simulink model "Simulation"  (Simulink 6.0)
settings: Solver=ode3  StartTime=0.0  StopTime=10  FixedStep=5e-3  RelTol=5e-3
values from neighbouring files (symbols this model uses):
  s = sqrt(1-rot(1,1)-rot(2,2)+rot(3,3))*2    [rot_to_quat2.m]
undefined symbols (not defined in the file or in its folder): sigbuilder_block
libraries: simulink x30, mblibv1 x15, aerolibtransform2 x4, vrlib x1
(part 2 of 2)

== system Simulation/Subsystem/Gestion Dynamique/Calcul orientation ==
  Erreur orientation : Inport  Port=1  LatchInput=off
  Orientation : Inport  Port=2  LatchInput=off
  Constant : Constant  Value=0
  Constant1 : Constant  Value=0
  Constant2 : Constant  Value=0
  Demux : Demux  Outputs=3
  Mux : Mux  Inputs=6
  Product : Product  RndMeth=Zero
  Product1 : Product  Multiplication=Matrix(*)  RndMeth=Zero
  Quaternion 2 AngleVecteur : Subsystem
  Quaternions to  Direction Cosine Matrix : aerolibtransform2/Quaternions to  Direction Cosine Matrix
  Reshape5 : simulink/Math Operations/Reshape  OutputDimensionality=1-D array  OutputDimensions=[1,1]
  Scope : Scope  NumInputPorts=2
      settings: YMin=-5~-5  YMax=5~5  SaveName=ScopeData11
  Ordres orientation : Outport
      settings: BusObject=perturbations
  wires:
  Mux/1 -> Reshape5/1
  Reshape5/1 -> Ordres orientation/1
  Constant/1 -> Mux/1
  Constant1/1 -> Mux/2
  Constant2/1 -> Mux/3
  Erreur orientation/1 -> Quaternion 2 AngleVecteur/1(Quaternion)
  Demux/1 -> Mux/4
  Demux/2 -> Mux/5
  Demux/3 -> Mux/6
  Product/1 -> Scope/2, Product1/2
  Quaternion 2 AngleVecteur/2(Vecteur) -> Product/2
  Quaternion 2 AngleVecteur/1(Angle) -> Product/1, Scope/1
  Quaternions to  Direction Cosine Matrix/1 -> Product1/1
  Product1/1 -> Demux/1
  Orientation/1 -> Quaternions to  Direction Cosine Matrix/1

== system Simulation/Subsystem/Gestion Dynamique/PID Attitude ==
  Entrée : Inport  Port=1  LatchInput=off
  Derivative : Derivative
  Derivative1 : Derivative
  Derivative2 : Derivative
  Gain : Gain  Gain=kp
  Gain1 : Gain  Gain=kd
  Gain2 : Gain  Gain=ki
  Gain3 : Gain  Gain=kdd
  Integrator : Integrator
  Reshape : simulink/Math Operations/Reshape  OutputDimensionality=1-D array  OutputDimensions=[1,1]
  Sum : Sum  Inputs=++++
  Sortie : Outport
      settings: BusObject=perturbations
  wires:
  Entrée/1 -> Gain/1
  Gain/1 -> Sum/2, Gain1/1, Gain2/1, Gain3/1
  Derivative/1 -> Sum/1
  Integrator/1 -> Sum/3
  Gain2/1 -> Integrator/1
  Gain1/1 -> Derivative/1
  Sum/1 -> Reshape/1
  Gain3/1 -> Derivative1/1
  Derivative1/1 -> Derivative2/1
  Derivative2/1 -> Sum/4
  Reshape/1 -> Sortie/1

== system Simulation/Subsystem/Gestion Dynamique/PID Position ==
  Entrée : Inport  Port=1  LatchInput=off
  Derivative : Derivative
  Derivative1 : Derivative
  Derivative2 : Derivative
  Gain : Gain  Gain=kp
  Gain1 : Gain  Gain=kd
  Gain2 : Gain  Gain=ki
  Gain3 : Gain  Gain=kdd
  Integrator : Integrator
  Reshape : simulink/Math Operations/Reshape  OutputDimensionality=1-D array  OutputDimensions=[1,1]
  Saturation : Saturate  UpperLimit=0.1  LowerLimit=-0.1
  Sum : Sum  Inputs=++++
  Sortie : Outport
      settings: BusObject=perturbations
  wires:
  Entrée/1 -> Gain/1
  Gain/1 -> Sum/2, Gain1/1, Gain2/1, Gain3/1
  Derivative/1 -> Sum/1
  Integrator/1 -> Saturation/1
  Gain2/1 -> Integrator/1
  Gain1/1 -> Derivative/1
  Sum/1 -> Reshape/1
  Gain3/1 -> Derivative1/1
  Derivative1/1 -> Derivative2/1
  Derivative2/1 -> Sum/4
  Reshape/1 -> Sortie/1
  Saturation/1 -> Sum/3

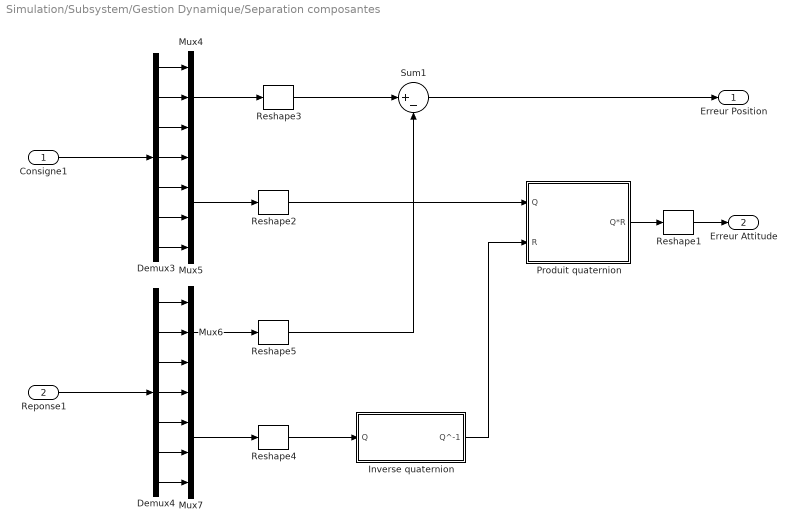
== system Simulation/Subsystem/Gestion Dynamique/Separation composantes ==
  Consigne1 : Inport  Port=1  LatchInput=off
  Reponse1 : Inport  Port=2  LatchInput=off
  Demux3 : Demux  Outputs=7
  Demux4 : Demux  Outputs=7
  Inverse quaternion : Subsystem
  Mux4 : Mux  Inputs=3
  Mux5 : Mux
  Mux6 : Mux  Inputs=3
  Mux7 : Mux
  Produit quaternion : Subsystem
  Reshape{1..5} (5 alike) : simulink/Math Operations/Reshape  OutputDimensionality=1-D array  OutputDimensions=[1,1]
  Sum1 : Sum  Inputs=|+-
  Erreur Position : Outport
      settings: BusObject=perturbations
  Erreur Attitude : Outport  Port=2
      settings: BusObject=perturbations
  wires:
  Consigne1/1 -> Demux3/1
  Demux3/4 -> Mux5/1
  Demux3/5 -> Mux5/2
  Demux3/6 -> Mux5/3
  Demux3/7 -> Mux5/4
  Demux3/3 -> Mux4/3
  Demux3/2 -> Mux4/2
  Demux3/1 -> Mux4/1
  Mux5/1 -> Reshape2/1
  Mux4/1 -> Reshape3/1
  Demux4/4 -> Mux7/1
  Demux4/5 -> Mux7/2
  Demux4/6 -> Mux7/3
  Demux4/7 -> Mux7/4
  Demux4/3 -> Mux6/3
  Demux4/2 -> Mux6/2
  Demux4/1 -> Mux6/1
  Reponse1/1 -> Demux4/1
  Mux7/1 -> Reshape4/1
  Mux6/1 -> Reshape5/1
  Reshape3/1 -> Sum1/1
  Reshape5/1 -> Sum1/2
  Sum1/1 -> Erreur Position/1
  Reshape4/1 -> Inverse quaternion/1(Q)
  Reshape2/1 -> Produit quaternion/1(Q)
  Inverse quaternion/1(Q^-1) -> Produit quaternion/2(R)
  Produit quaternion/1(Q*R) -> Reshape1/1
  Reshape1/1 -> Erreur Attitude/1

== system Simulation/Subsystem/Gestion Dynamique/Separation composantes1 ==
  Entree : Inport  Port=1  LatchInput=off
  Demux1 : Demux  Outputs=7
  Mux : Mux  Inputs=3
  Mux1 : Mux
  Reshape : simulink/Math Operations/Reshape  OutputDimensionality=1-D array  OutputDimensions=[1,1]
  Reshape1 : simulink/Math Operations/Reshape  OutputDimensionality=1-D array  OutputDimensions=[1,1]
  Position : Outport
      settings: BusObject=perturbations
  Orientation : Outport  Port=2
      settings: BusObject=perturbations
  wires:
  Entree/1 -> Demux1/1
  Demux1/4 -> Mux1/1
  Demux1/5 -> Mux1/2
  Demux1/6 -> Mux1/3
  Demux1/7 -> Mux1/4
  Demux1/3 -> Mux/3
  Demux1/2 -> Mux/2
  Demux1/1 -> Mux/1
  Mux1/1 -> Reshape/1
  Mux/1 -> Reshape1/1
  Reshape/1 -> Orientation/1
  Reshape1/1 -> Position/1

== system Simulation/Subsystem/Gestion Dynamique/Sommation ordres ==
  Ordres position : Inport  Port=1  LatchInput=off
  Ordres orientation : Inport  Port=2  LatchInput=off
  Sum : Sum
  Ordres : Outport
      settings: BusObject=perturbations
  wires:
  Ordres orientation/1 -> Sum/2
  Sum/1 -> Ordres/1
  Ordres position/1 -> Sum/1

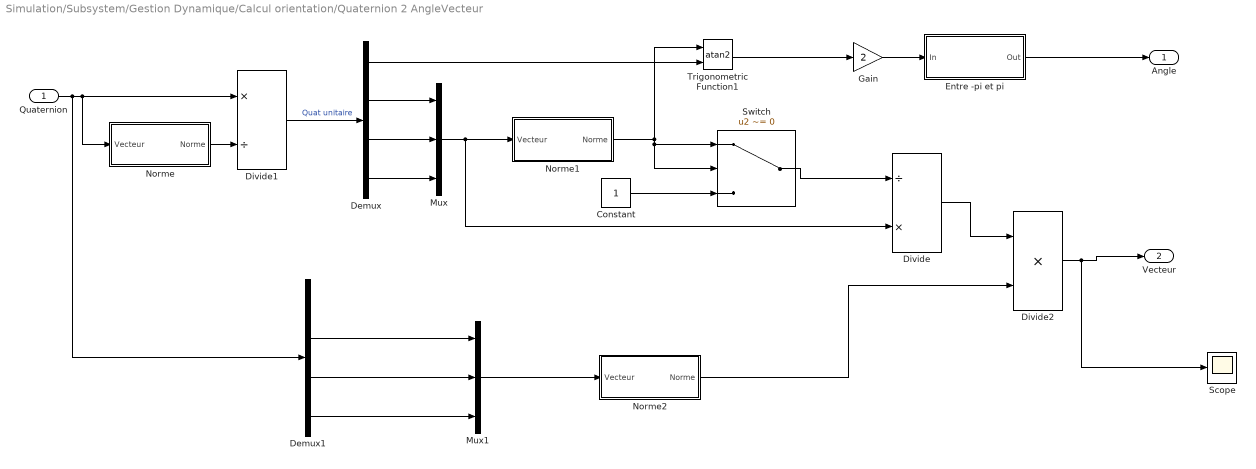
== system Simulation/Subsystem/Gestion Dynamique/Calcul orientation/Quaternion 2 AngleVecteur ==
  Quaternion : Inport  Port=1  LatchInput=off
  Constant : Constant
  Demux : Demux
  Demux1 : Demux
  Divide : Product  Inputs=/*  OutScaling=2^-10
  Divide1 : Product  Inputs=*/  OutScaling=2^-10
  Divide2 : Product  Inputs=**  OutScaling=2^-10
  Entre -pi et pi : Subsystem  mask{ordre=2}
  Gain : Gain  Gain=2
  Mux : Mux  Inputs=3
  Mux1 : Mux  Inputs=3
  Norme : Subsystem  mask{ordre=2}
      mask Display: text(0.3,0.5,strcat('Norme',get_param(gcb, 'ordre')));
  Norme1 : Subsystem  mask{ordre=2}
      mask Display: text(0.3,0.5,strcat('Norme',get_param(gcb, 'ordre')));
  Norme2 : Subsystem  mask{ordre=2}
      mask Display: text(0.3,0.5,strcat('Norme',get_param(gcb, 'ordre')));
  Scope : Scope
      settings: SaveName=ScopeData10
  Switch : Switch  Criteria=u2 ~= 0
  Trigonometric Function1 : Trigonometry  Operator=atan2
  Angle : Outport
  Vecteur : Outport  Port=2
  wires:
  Quaternion/1 -> Divide1/1, Norme/1(Vecteur), Demux1/1
  Trigonometric Function1/1 -> Gain/1
  Norme/1(Norme) -> Divide1/2
  Divide1/1 -> Demux/1  "Quat unitaire"
  Mux/1 -> Norme1/1(Vecteur), Divide/2
  Demux/2 -> Mux/1
  Demux/3 -> Mux/2
  Demux/4 -> Mux/3
  Norme1/1(Norme) -> Trigonometric Function1/1, Switch/2, Switch/1
  Demux/1 -> Trigonometric Function1/2
  Switch/1 -> Divide/1
  Constant/1 -> Switch/3
  Entre -pi et pi/1(Out) -> Angle/1
  Gain/1 -> Entre -pi et pi/1(In)
  Demux1/2 -> Mux1/1
  Demux1/3 -> Mux1/2
  Demux1/4 -> Mux1/3
  Mux1/1 -> Norme2/1(Vecteur)
  Divide/1 -> Divide2/1
  Norme2/1(Norme) -> Divide2/2
  Divide2/1 -> Vecteur/1, Scope/1

== system Simulation/Subsystem/Gestion Dynamique/Separation composantes/Inverse quaternion ==
  Q : Inport  Port=1  LatchInput=off
  Gain : Gain  Gain=[1 -1 -1 -1]
  Q^-1 : Outport
  wires:
  Q/1 -> Gain/1
  Gain/1 -> Q^-1/1

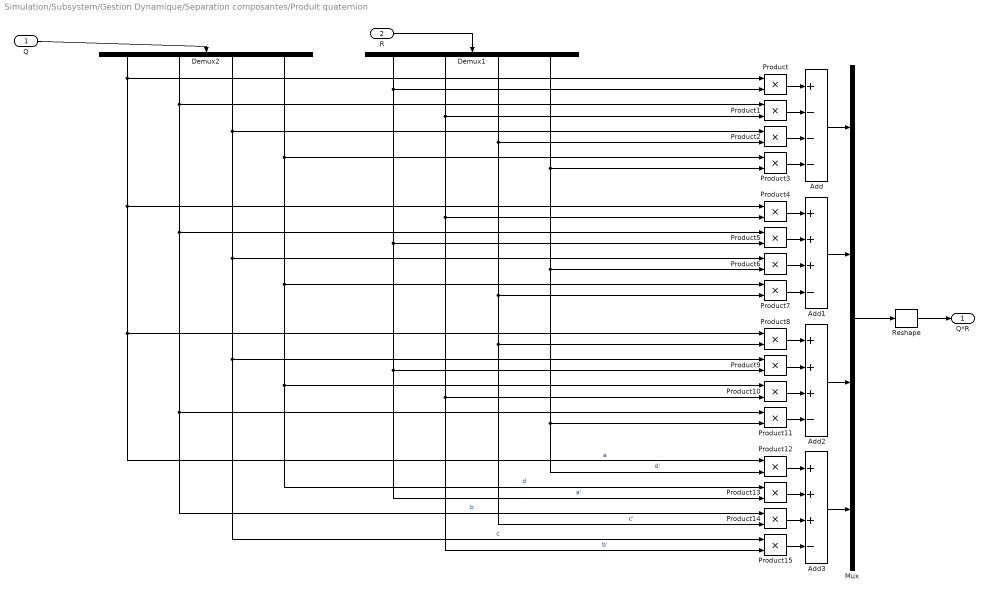
== system Simulation/Subsystem/Gestion Dynamique/Separation composantes/Produit quaternion ==
  Q : Inport  Port=1  LatchInput=off
  R : Inport  Port=2  LatchInput=off
  Add : Sum  Inputs=+---  OutScaling=2^-10
  Add1 : Sum  Inputs=+++-  OutScaling=2^-10
  Add2 : Sum  Inputs=+++-  OutScaling=2^-10
  Add3 : Sum  Inputs=+++-  OutScaling=2^-10
  Demux1 : Demux  Orientation=down
  Demux2 : Demux  Orientation=down
  Mux : Mux
  Product{,1..15} (16 alike) : Product  RndMeth=Zero
  Reshape : simulink/Math Operations/Reshape  OutputDimensionality=1-D array  OutputDimensions=[1,1]
  Q*R : Outport
  wires:
  R/1 -> Demux1/1
  Q/1 -> Demux2/1
  Mux/1 -> Reshape/1
  Reshape/1 -> Q*R/1
  Demux2/1 -> Product/1, Product4/1, Product8/1, Product12/1  "a"
  Add/1 -> Mux/1
  Add1/1 -> Mux/2
  Add2/1 -> Mux/3
  Add3/1 -> Mux/4
  Product3/1 -> Add/4
  Product2/1 -> Add/3
  Product1/1 -> Add/2
  Product/1 -> Add/1
  Product7/1 -> Add1/4
  Product6/1 -> Add1/3
  Product5/1 -> Add1/2
  Product4/1 -> Add1/1
  Product11/1 -> Add2/4
  Product10/1 -> Add2/3
  Product9/1 -> Add2/2
  Product8/1 -> Add2/1
  Product15/1 -> Add3/4
  Product14/1 -> Add3/3
  Product13/1 -> Add3/2
  Product12/1 -> Add3/1
  Demux2/2 -> Product1/1, Product5/1, Product11/1, Product14/1  "b"
  Demux2/3 -> Product2/1, Product6/1, Product9/1, Product15/1  "c"
  Demux2/4 -> Product3/1, Product7/1, Product10/1, Product13/1  "d"
  Demux1/1 -> Product/2, Product5/2, Product9/2, Product13/2  "a'"
  Demux1/2 -> Product1/2, Product4/2, Product10/2, Product15/2  "b'"
  Demux1/3 -> Product2/2, Product7/2, Product8/2, Product14/2  "c'"
  Demux1/4 -> Product3/2, Product6/2, Product11/2, Product12/2  "d'"

== system Simulation/Subsystem/Gestion Dynamique/Calcul orientation/Quaternion 2 AngleVecteur/Entre -pi et pi ==
  In : Inport  Port=1  LatchInput=off
  Constant1 : Constant  Value=pi
  Constant2 : Constant  Value=2*pi
  Constant3 : Constant  Value=pi
  Math Function3 : Math  Operator=mod  SaturateOnIntegerOverflow=on
  Subtract : Sum  OutScaling=2^-10
  Subtract1 : Sum  Inputs=+-  OutScaling=2^-10
  Out : Outport
  wires:
  Subtract/1 -> Math Function3/1
  Constant2/1 -> Math Function3/2
  In/1 -> Subtract/1
  Constant1/1 -> Subtract/2
  Math Function3/1 -> Subtract1/1
  Constant3/1 -> Subtract1/2
  Subtract1/1 -> Out/1

== system Simulation/Subsystem/Gestion Dynamique/Calcul orientation/Quaternion 2 AngleVecteur/Norme ==
  Vecteur : Inport  Port=1  LatchInput=off
  Constant1 : Constant  Value=ordre
  Math Function : Math  Operator=pow  SaturateOnIntegerOverflow=on
  Math Function1 : Math  Operator=reciprocal  SaturateOnIntegerOverflow=on
  Math Function2 : Math  Operator=pow  SaturateOnIntegerOverflow=on
  Sum of Elements : Sum  Inputs=+  OutScaling=2^-10
  Norme : Outport
  wires:
  Math Function/1 -> Sum of Elements/1
  Vecteur/1 -> Math Function/1
  Constant1/1 -> Math Function/2, Math Function1/1
  Math Function1/1 -> Math Function2/2
  Sum of Elements/1 -> Math Function2/1
  Math Function2/1 -> Norme/1

== system Simulation/Subsystem/Gestion Dynamique/Calcul orientation/Quaternion 2 AngleVecteur/Norme1 ==
  Vecteur : Inport  Port=1  LatchInput=off
  Constant1 : Constant  Value=ordre
  Math Function : Math  Operator=pow  SaturateOnIntegerOverflow=on
  Math Function1 : Math  Operator=reciprocal  SaturateOnIntegerOverflow=on
  Math Function2 : Math  Operator=pow  SaturateOnIntegerOverflow=on
  Sum of Elements : Sum  Inputs=+  OutScaling=2^-10
  Norme : Outport
  wires:
  Math Function/1 -> Sum of Elements/1
  Vecteur/1 -> Math Function/1
  Constant1/1 -> Math Function/2, Math Function1/1
  Math Function1/1 -> Math Function2/2
  Sum of Elements/1 -> Math Function2/1
  Math Function2/1 -> Norme/1

== system Simulation/Subsystem/Gestion Dynamique/Calcul orientation/Quaternion 2 AngleVecteur/Norme2 ==
  Vecteur : Inport  Port=1  LatchInput=off
  Constant1 : Constant  Value=ordre
  Math Function : Math  Operator=pow  SaturateOnIntegerOverflow=on
  Math Function1 : Math  Operator=reciprocal  SaturateOnIntegerOverflow=on
  Math Function2 : Math  Operator=pow  SaturateOnIntegerOverflow=on
  Sum of Elements : Sum  Inputs=+  OutScaling=2^-10
  Norme : Outport
  wires:
  Math Function/1 -> Sum of Elements/1
  Vecteur/1 -> Math Function/1
  Constant1/1 -> Math Function/2, Math Function1/1
  Math Function1/1 -> Math Function2/2
  Sum of Elements/1 -> Math Function2/1
  Math Function2/1 -> Norme/1
